simulink model "HILSimulation2024a"  (R2024a)
settings: Solver=FixedStepAuto  StartTime=0.0  StopTime=inf  FixedStep=0.05  RelTol=1e-3
model workspace (MAT data in the model file):
  NumRxValues = 10
  NumTxVariables = 4
values from neighbouring files (symbols this model uses):
  DryMass = 3    [FlightPathGeneration.m]
  LaunchSitePressure = PlanMeta(7)    [FlightAnalysis.m]    (also in FlightPathGeneration.m = 101325; TargetApogeeSelection.m = 101325)
  LaunchSiteTemperature = PlanMeta(6)    [FlightAnalysis.m]    (also in FlightPathGeneration.m = 288.15; TargetApogeeSelection.m = 288.15)
  MinimumDragArea = 0.0025    [FlightPathGeneration.m]    (also in TargetApogeeSelection.m)
undefined symbols (not defined in the file or in its folder): f
libraries: instrumentlib x2
settings Model: Creator=natha  LastModifiedBy=natha

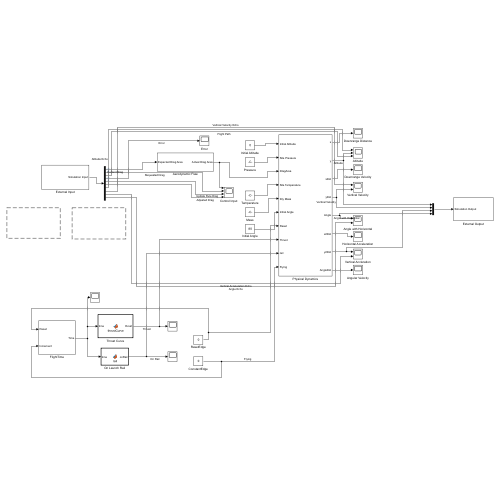
[thumbnail: Simulink's stored preview of the top-level diagram]
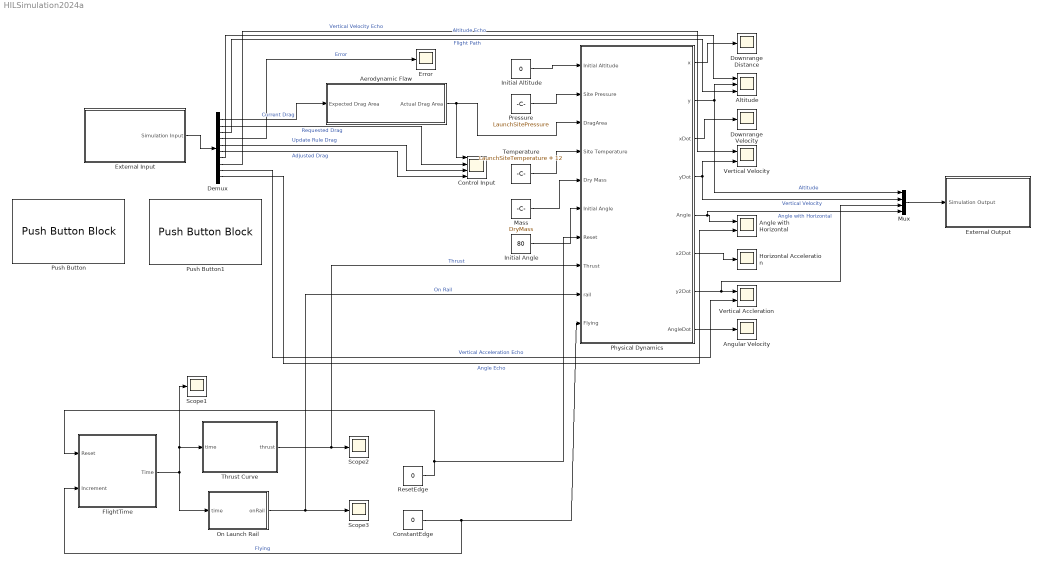
== system HILSimulation2024a ==
  Aerodynamic Flaw : Subsystem
  Altitude : Scope  NumInputPorts=3
  Angle with Horizontal : Scope  NumInputPorts=2
  Angular Velocity : Scope
  ConstantEdge : Constant  Value=0
  Control Input : Scope  NumInputPorts=4
  Demux : Demux  Outputs=NumRxValues
  Downrange Distance : Scope
  Downrange Velocity : Scope
  Error : Scope
  External Input : Subsystem
  External Output : Subsystem
  FlightTime : Subsystem
  Horizontal Acceleration : Scope
  Initial Altitude : Constant  Value=0
  Initial Angle : Constant  Value=80
  Mass : Constant  Value=DryMass
  Mux : Mux  Inputs=NumTxVariables
  On Launch Rail : MATLAB Function  TreatAsAtomicUnit=on
  Physical Dynamics : Subsystem
  Pressure : Constant  Value=LaunchSitePressure
  Push Button : PushButtonBlock  ButtonText=Reset  OffValue=0.000000
  Push Button1 : PushButtonBlock  ButtonText=Launch  ButtonType=Latch  OffValue=0.000000
  ResetEdge : Constant  Value=0
  Scope1 : Scope
  Scope2 : Scope
  Scope3 : Scope
  Temperature : Constant  Value=LaunchSiteTemperature + 12
  Thrust Curve : MATLAB Function  TreatAsAtomicUnit=on
  Vertical Accleration : Scope  NumInputPorts=2
  Vertical Velocity : Scope  NumInputPorts=2
  wires:
  External Input/1(Simulation Input) -> Demux/1
  Mux/1 -> External Output/1(Simulation Output)
  Initial Altitude/1 -> Physical Dynamics/1(Initial Altitude)
  Pressure/1 -> Physical Dynamics/2(Site Pressure)
  Temperature/1 -> Physical Dynamics/4(Site Temperature)
  Mass/1 -> Physical Dynamics/5(Dry Mass)
  Physical Dynamics/2(y) -> Altitude/2, Mux/1  "Altitude"
  Physical Dynamics/4(yDot) -> Vertical Velocity/2, Mux/2  "Vertical Velocity"
  Physical Dynamics/5(Angle) -> Mux/4, Angle with Horizontal/1  "Angle with Horizontal"
  Physical Dynamics/1(x) -> Downrange Distance/1
  Physical Dynamics/3(xDot) -> Downrange Velocity/1
  Physical Dynamics/6(x2Dot) -> Horizontal Acceleration/1
  Physical Dynamics/8(AngleDot) -> Angular Velocity/1
  Physical Dynamics/7(y2Dot) -> Mux/3, Vertical Accleration/1
  Demux/7 -> Altitude/1  "Altitude Echo"
  Demux/8 -> Vertical Velocity/1  "Vertical Velocity Echo"
  Demux/5 -> Control Input/3  "Update Rule Drag"
  Demux/6 -> Control Input/4  "Adjusted Drag"
  Demux/3 -> Altitude/3  "Flight Path"
  Demux/4 -> Error/1  "Error"
  Initial Angle/1 -> Physical Dynamics/6(Initial Angle)
  ResetEdge/1 -> FlightTime/1(Reset), Physical Dynamics/7(Reset)
  FlightTime/1(Time) -> Scope1/1, Thrust Curve/1(time), On Launch Rail/1(time)
  Thrust Curve/1(thrust) -> Physical Dynamics/8(Thrust), Scope2/1  "Thrust"
  On Launch Rail/1(onRail) -> Scope3/1, Physical Dynamics/9(rail)  "On Rail"
  ConstantEdge/1 -> FlightTime/2(Increment), Physical Dynamics/10(Flying)  "Flying"
  Demux/9 -> Vertical Accleration/2  "Vertical Acceleration Echo"
  Demux/10 -> Angle with Horizontal/2  "Angle Echo"
  Demux/2 -> Control Input/2  "Requested Drag"
  Demux/1 -> Aerodynamic Flaw/1(Expected Drag Area)  "Current Drag"
  Aerodynamic Flaw/1(Actual Drag Area) -> Control Input/1, Physical Dynamics/3(DragArea)

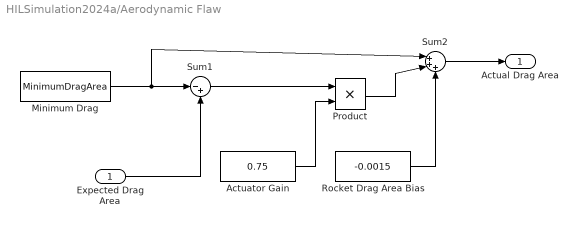
== system HILSimulation2024a/Aerodynamic Flaw ==
  Expected Drag Area : Inport
  Actuator Gain : Constant  Value=0.75
  Minimum Drag : Constant  Value=MinimumDragArea
  Product : Product
  Rocket Drag Area Bias : Constant  Value=-0.0015
  Sum1 : Sum  Inputs=|-+
  Sum2 : Sum  Inputs=|+++
  Actual Drag Area : Outport
  wires:
  Minimum Drag/1 -> Sum2/1, Sum1/1
  Expected Drag Area/1 -> Sum1/2
  Sum1/1 -> Product/1
  Actuator Gain/1 -> Product/2
  Sum2/1 -> Actual Drag Area/1
  Product/1 -> Sum2/2
  Rocket Drag Area Bias/1 -> Sum2/3

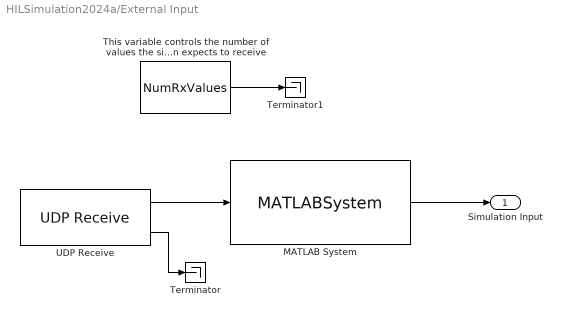
== system HILSimulation2024a/External Input ==
  MATLAB System : MATLABSystem  System=BytesToFloats  NumValues=NumRxValues  SimulateUsing=Code generation
      mask Type: BytesToFloats
      mask Display:
      | disp('BytesToFloats');
      | port_label('input',1,'bytes');
      | port_label('output',1,'floatValues');
  Terminator : Terminator
  Terminator1 : Terminator
  This variable controls the number of values the simulation expects to receive : Constant  Value=NumRxValues
  UDP Receive : instrumentlib/UDP Receive  LocalAddress=127.0.0.1  LocalPort=25000  EnablePortSharing=off  Host=localhost  Port=25001  GetLatestData=on  DataSize=[ 1, 8*NumRxValues ]  DataType=uint8  ASCIIFormatting=%f,  Terminator=LF  CustomTerminator=10  ByteOrder=big-endian  EnableBlockingMode=off  Timeout=10  SampleTime=0.05  SimulateUsing=Interpreted execution
  Simulation Input : Outport
  wires:
  UDP Receive/1 -> MATLAB System/1
  MATLAB System/1 -> Simulation Input/1
  UDP Receive/2 -> Terminator/1
  This variable controls the number of values the simulation expects to receive/1 -> Terminator1/1

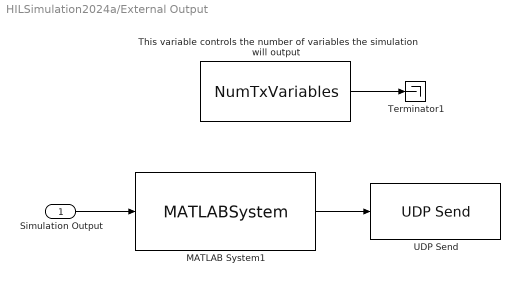
== system HILSimulation2024a/External Output ==
  Simulation Output : Inport
  MATLAB System1 : MATLABSystem  System=FloatsToBytes  NumValues=NumTxVariables  SimulateUsing=Code generation
      mask Type: FloatsToBytes
      mask Display:
      | disp('FloatsToBytes');
      | port_label('input',1,'floatValues');
      | port_label('output',1,'bytes');
  Terminator1 : Terminator
  This variable controls the number of variables the simulation will output : Constant  Value=NumTxVariables
  UDP Send : instrumentlib/UDP Send  Host=127.0.0.1  Port=25001  LocalAddress=127.0.0.1  LocalPort=25000  EnablePortSharing=off  OutputDatagramPacketSize=8 * NumTxVariables  ByteOrder=big-endian  EnableBlockingMode=off  SimulateUsing=Interpreted execution
  wires:
  MATLAB System1/1 -> UDP Send/1
  Simulation Output/1 -> MATLAB System1/1
  This variable controls the number of variables the simulation will output/1 -> Terminator1/1

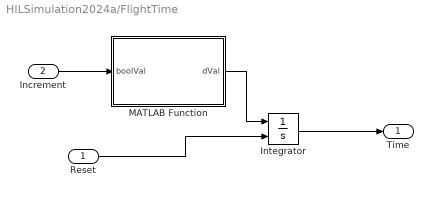
== system HILSimulation2024a/FlightTime ==
  Reset : Inport
  Increment : Inport  Port=2
  Integrator : Integrator  ExternalReset=rising
  MATLAB Function : MATLAB Function  TreatAsAtomicUnit=on
  Time : Outport
  wires:
  Integrator/1 -> Time/1
  Reset/1 -> Integrator/2
  Increment/1 -> MATLAB Function/1(boolVal)
  MATLAB Function/1(dVal) -> Integrator/1

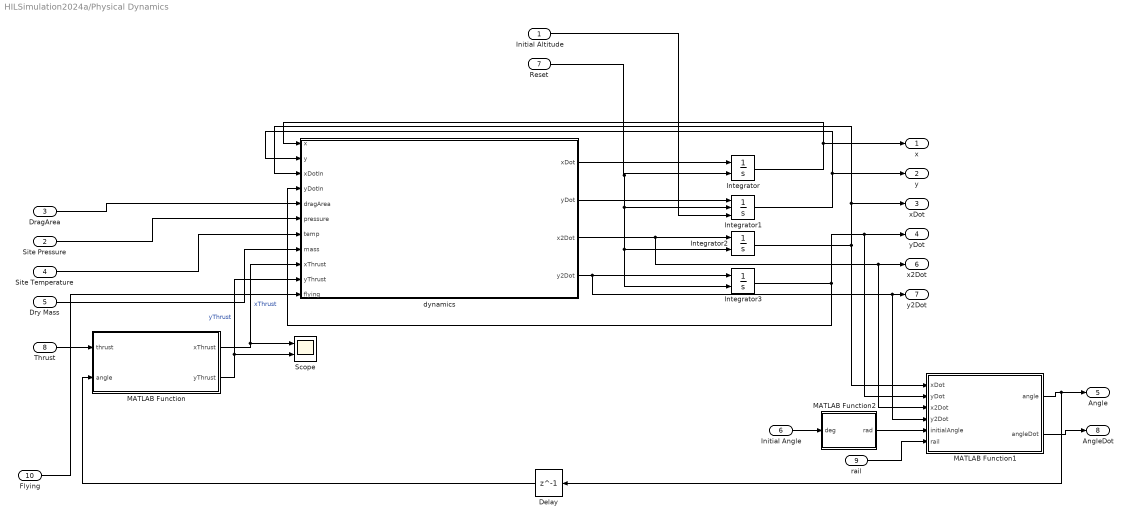
== system HILSimulation2024a/Physical Dynamics ==
  Initial Altitude : Inport
  Site Pressure : Inport  Port=2
  DragArea : Inport  Port=3
  Site Temperature : Inport  Port=4
  Dry Mass : Inport  Port=5
  Initial Angle : Inport  Port=6
  Reset : Inport  Port=7
  Thrust : Inport  Port=8
  rail : Inport  Port=9
  Flying : Inport  Port=10
  Delay : Delay  DelayLength=1  InputProcessing=Columns as channels (frame based)
  Integrator : Integrator  ExternalReset=rising
  Integrator1 : Integrator  ExternalReset=rising  InitialConditionSource=external
  Integrator2 : Integrator  ExternalReset=rising
  Integrator3 : Integrator  ExternalReset=rising
  MATLAB Function : MATLAB Function  TreatAsAtomicUnit=on
  MATLAB Function1 : MATLAB Function  TreatAsAtomicUnit=on
  MATLAB Function2 : MATLAB Function  TreatAsAtomicUnit=on
  Scope : Scope  NumInputPorts=2
  dynamics : MATLAB Function  TreatAsAtomicUnit=on
  x : Outport
  y : Outport  Port=2
  xDot : Outport  Port=3
  yDot : Outport  Port=4
  Angle : Outport  Port=5
  x2Dot : Outport  Port=6
  y2Dot : Outport  Port=7
  AngleDot : Outport  Port=8
  wires:
  dynamics/1(xDot) -> Integrator/1
  Integrator2/1 -> MATLAB Function1/1(xDot), xDot/1, dynamics/3(xDotIn)
  dynamics/4(y2Dot) -> Integrator3/1, MATLAB Function1/4(y2Dot), y2Dot/1
  dynamics/2(yDot) -> Integrator1/1
  dynamics/3(x2Dot) -> MATLAB Function1/3(x2Dot), x2Dot/1, Integrator2/1
  DragArea/1 -> dynamics/5(dragArea)
  Integrator3/1 -> dynamics/4(yDotIn), MATLAB Function1/2(yDot), yDot/1
  Integrator/1 -> x/1, dynamics/1(x)
  Integrator1/1 -> y/1, dynamics/2(y)
  Dry Mass/1 -> dynamics/8(mass)
  Site Pressure/1 -> dynamics/6(pressure)
  Initial Altitude/1 -> Integrator1/3
  Site Temperature/1 -> dynamics/7(temp)
  Reset/1 -> Integrator3/2, Integrator2/2, Integrator1/2, Integrator/2
  MATLAB Function/1(xThrust) -> Scope/1, dynamics/9(xThrust)  "xThrust"
  MATLAB Function/2(yThrust) -> Scope/2, dynamics/10(yThrust)  "yThrust"
  Thrust/1 -> MATLAB Function/1(thrust)
  MATLAB Function1/2(angleDot) -> AngleDot/1
  MATLAB Function1/1(angle) -> Delay/1, Angle/1
  Initial Angle/1 -> MATLAB Function2/1(deg)
  rail/1 -> MATLAB Function1/6(rail)
  Flying/1 -> dynamics/11(flying)
  Delay/1 -> MATLAB Function/2(angle)
  MATLAB Function2/1(rad) -> MATLAB Function1/5(initialAngle)

== matlab function HILSimulation2024a/Thrust Curve ==
  data: time input; thrust output
function thrust = thrustCurve(time)
if(time < 1.1 && time > 0)
    thrust = 140;
else
    thrust = 0;
end

== matlab function HILSimulation2024a/Physical Dynamics/dynamics ==
  data: xDot output; yDot output; x2Dot output; y2Dot output; x input; y input; xDotIn input; yDotIn input; dragArea input; pressure input; temp input; mass input; xThrust input; yThrust input; flying input
function [xDot,yDot, x2Dot, y2Dot] = dynamics(x, y, xDotIn, yDotIn, dragArea, pressure, temp, mass, xThrust, yThrust, flying)
%constants---
g = 9.8;
%------------
x;
xDot = xDotIn;
yDot = yDotIn;
if(flying)
    x2Dot = -1/2/mass * densityFromAltitude(y, pressure, temp) * dragArea * sqrt(xDot * xDot + yDot * yDot) * xDot + xThrust;
    y2Dot = -1/2/mass * densityFromAltitude(y, pressure, temp) * dragArea * sqrt(xDot * xDot + yDot * yDot) * yDot - g + yThrust;
else
    x2Dot = 0;
    y2Dot = 0;
end
end


function density = densityFromAltitude(altitude, p0, T0)
    % Constants
    L = 0.0065;      % K/m temperature lapse rate
    g = 9.80665;     % m/s^2 gravitational constant
    R = 8.31446;     % J/(mol*K) Ideal gas constant
    M = 0.0289652;   % kg/mol Molar mass of air
    density = p0*M/(R*T0)*(1-L*altitude/T0).^(g*M/(R*L)-1);
end

== matlab function HILSimulation2024a/Physical Dynamics/MATLAB Function ==
  data: thrust input; xThrust output; angle input; yThrust output
function [xThrust, yThrust] = thrustComponents(thrust, angle)
    xThrust = thrust * cos(angle);
    yThrust = thrust * sin(angle);
end

== matlab function HILSimulation2024a/Physical Dynamics/MATLAB Function1 ==
  data: xDot input; angle output; yDot input; x2Dot input; y2Dot input; angleDot output; initialAngle input; rail input
function [angle, angleDot] = angles(xDot, yDot, x2Dot, y2Dot, initialAngle, rail)
    if(rail)
        angle = initialAngle;
        angleDot = 0;
    else
        angle = atan(yDot/xDot);
        angleDot = (y2Dot * xDot - yDot * x2Dot) / (xDot * xDot + yDot * yDot);
    end
end

== matlab function HILSimulation2024a/On Launch Rail ==
  data: time input; onRail output
function onRail = rail(time)
if(time < 0.5)
    onRail = 1;
else
    onRail = 0;
end

== matlab function HILSimulation2024a/FlightTime/MATLAB Function ==
  data: boolVal input; dVal output
function dVal = cast(boolVal)
if(boolVal)
    dVal = 1;
else
    dVal = 0;
end

== matlab function HILSimulation2024a/Physical Dynamics/MATLAB Function2 ==
  data: deg input; rad output
function rad = toRad(deg)
    rad = deg * pi / 180;
end
